simulink model "multiRobotSoccer"  (R2022b)
settings: Solver=FixedStepAuto  StartTime=0.0  StopTime=inf  FixedStep=sampleTime  RelTol=1e-3
PreLoadFcn:
  | robotSoccerParams;
values from neighbouring files (symbols this model uses):
  angThresh = pi/16    (= 0.196349540849)    [robotSoccerParams.m]
  attackerKickSpeed = 3    [robotSoccerParams.m]
  attackerMaxGoalDist = 10    [robotSoccerParams.m]
  attackerMinGoalDist = 5    [robotSoccerParams.m]
  awayGoalPosition = [fieldLimitsX(2) mean(fieldLimitsY)]    [robotSoccerParams.m]
  ballAngleNoise = pi/24    (= 0.1308996939)    [robotSoccerParams.m]
  ballThresh = robotRadius + 0.3    (= 1.1)    [robotSoccerParams.m]
  ballVelNoise = 0.5    [robotSoccerParams.m]
  defenderAwayPoses = [82 28.5 pi ... (first row only)    [robotSoccerParams.m]
  defenderHomePoses = [10 28.5 0 ... (first row only)    [robotSoccerParams.m]
  defenderKickSpeed = 5    [robotSoccerParams.m]
  distThresh = 1    [robotSoccerParams.m]
  dribbleKickSpeed = 2    [robotSoccerParams.m]
  dribbleTime = 25    [robotSoccerParams.m]
  fieldCenter = [mean(fieldLimitsX) mean(fieldLimitsY)]    [robotSoccerParams.m]
  fieldLimitsX = [0 92]    [robotSoccerParams.m]
  fieldLimitsY = [0 47]    [robotSoccerParams.m]
  goalkeeperKickSpeed = 10    [robotSoccerParams.m]
  goalkeeperPoses = [ 2 23.5 0 ... (first row only)    [robotSoccerParams.m]
  goalPosts = [ 0 33 2 ... (first row only)    [robotSoccerParams.m]
  goalThresh = 20    [robotSoccerParams.m]
  homeGoalPosition = [fieldLimitsX(1) mean(fieldLimitsY)]    [robotSoccerParams.m]
  initBallPos = fieldCenter    [robotSoccerParams.m]
  initGameState = struct('possession',0,                         'state',GameState.InPlay,                         'score',[0;0])    [robotSoccerParams.m]
  numRobots = 8    [robotSoccerParams.m]
  objColors = [0 0.75 0; 1 0 0; 0 0 1]    [robotSoccerParams.m]
  objMarkers = 'o^^'    [robotSoccerParams.m]
  outOfBoundsDist = 2    [robotSoccerParams.m]
  robotDetectorMaxHits = 5    [robotSoccerParams.m]
  robotRadius = 0.8    [robotSoccerParams.m]
undefined symbols (not defined in the file or in its folder): DiscIntNeverNeededParam, ObjectType
libraries: soccerRobotLib x8
(part 2 of 2)

== stateflow chart multiRobotSoccer/Robot Behavior/For Each Subsystem (Iterates through all robots)/SoccerBehavior ==
  settings: updateMethod=DISCRETE  sampleTime=sampleTime
  state ExecuteBehavior [parallel]
    en,du:
    prevRole = behavior.role;
    settings: executionOrder=1
    state Attack
      % Attack logic: Go to the ball, carry it near the goal, and shoot!
      en:
      if behavior.team == 1
      goalPose = [awayGoalPosition';0];
      else
      goalPose = [homeGoalPosition';pi];
      end
      state GoToBall
        en:
        commands.action = RobotAction.HoldBall;
        en,du:
        [ballRange,ballAngle] = detectBall(sensors.detections);
        commands.robotVelocity = trackDetection(ballRange,ballAngle);
      state KickBall
        en:
        commands.action = RobotAction.KickBall;
        commands.robotVelocity = [0;0;0];
        commands.ballVelocity = attackerKickSpeed;
      state GoToGoal
        en:
        commands.action = RobotAction.HoldBall;
        en,du:
        [goalDistance,goalAngle] = calcBearing(goalPose);
        commands.robotVelocity = goToPose(goalPose);
      state Dribble
        %Dribble the ball if held for too long
        en:
        commands.action = RobotAction.KickBall;
        commands.ballVelocity = dribbleKickSpeed;
      state BackUp
        % Move out of goal if too close
        en:
        commands.action = RobotAction.HoldBall;
        en,du:
        commands.robotVelocity = goToPose([fieldCenter';pi/2]);
      (default) -> GoToBall
      GoToBall -> ExecuteBehavior.Attack.GoToGoal : [sensors.ballHeld]
      ExecuteBehavior.Attack.KickBall -> GoToBall : [after(1,sec)]
      ExecuteBehavior.Attack.GoToGoal -> ExecuteBehavior.Attack.KickBall [order 2] : [goalDistance <= goalThresh && ...
          |  abs(goalAngle) < angThresh]
      ExecuteBehavior.Attack.GoToGoal -> Dribble [order 3] : [after(dribbleTime,sec)]
      Dribble -> ExecuteBehavior.Attack.GoToGoal : [after(0.5,sec)]
      ExecuteBehavior.Attack.GoToGoal -> BackUp [order 1] : [abs(sensors.pose(1) - goalPose(1)) < ...
          | attackerMinGoalDist]
      BackUp -> ExecuteBehavior.Attack.GoToGoal : [abs(sensors.pose(1) - goalPose(1)) > ...
          | attackerMaxGoalDist]
    state Defend
      % Defense logic: If own team has ball possession, go to the goal. Else, chase after the ball.
      state DefensiveActions
        en,du:
        ballRange = detectBall(sensors.detections);
        state DefendGoal
          en:
          commands.action = RobotAction.HoldBall;
          goalPose = behavior.formationPose;
          en,du:
          commands.robotVelocity = goToPose(goalPose);
        state ChaseBall
          en,du:
          if behavior.possessingTeam == 0
          commands.action = RobotAction.HoldBall;
          else
          commands.action = RobotAction.DoNothing;
          end
          [ballRange,ballAngle] = detectBall(sensors.detections);
          commands.robotVelocity = trackDetection(ballRange,ballAngle);
        (default) -> ExecuteBehavior.Defend.DefensiveActions.DefendGoal
        ExecuteBehavior.Defend.DefensiveActions.ChaseBall -> ExecuteBehavior.Defend.DefensiveActions.DefendGoal : [behavior.possessingTeam == behavior.team]
        ExecuteBehavior.Defend.DefensiveActions.DefendGoal -> ExecuteBehavior.Defend.DefensiveActions.ChaseBall : [behavior.possessingTeam == 0 ...
            |  && distToOwnGoal < diff(fieldLimitsX)/2 && ...
            |  ballRange < diff(fieldLimitsX)/1.5 && ballRange > 0]
      state TurnToGoal
        en:
        if behavior.team == 1
        goalPose = [awayGoalPosition';0];
        else
        goalPose = [homeGoalPosition';pi];
        end
        en,du:
        commands.action = RobotAction.HoldBall;
        [commands.robotVelocity,isdone] = turnToPoint(goalPose);
      state KickBall
        en:
        commands.action = RobotAction.KickBall;
        commands.robotVelocity = [0;0;0];
        commands.ballVelocity = defenderKickSpeed;
      state dist = distToOwnGoal [function]
        (default) -> (junction 441)
        (junction 441) -> (junction 444) [order 1] : [behavior.team == 1]
        (junction 441) -> (junction 448) [order 2] : {dist = calcBearing(awayGoalPosition');}
        (junction 444) -> (junction 446) : {dist = calcBearing(homeGoalPosition');}
        (junction 446) -> (junction 448)
      (default) -> ExecuteBehavior.Defend.DefensiveActions
      ExecuteBehavior.Defend.DefensiveActions -> ExecuteBehavior.Defend.TurnToGoal : [sensors.ballHeld]
      ExecuteBehavior.Defend.TurnToGoal -> ExecuteBehavior.Defend.KickBall : [isdone || after(10,sec)]
      ExecuteBehavior.Defend.KickBall -> ExecuteBehavior.Defend.DefensiveActions : [after(1,sec)]
    state Defend1
      % Defense logic: If own team has ball possession, go to the goal. Else, chase after the ball.
      state DefensiveActions
        en,du:
        ballRange = detectBall(sensors.detections);
        state DefendGoal
          en:
          commands.action = RobotAction.HoldBall;
          goalPose = behavior.formationPose;
          en,du:
          if behavior.possessingTeam == 0
          commands.action = RobotAction.HoldBall;
          else
          commands.action = RobotAction.DoNothing;
          end
          [ballRange,ballAngle] = detectBall(sensors.detections);
          commands.robotVelocity = trackDetection(ballRange,ballAngle);
        state ChaseBall
          en,du:
          if behavior.possessingTeam == 0
          commands.action = RobotAction.HoldBall;
          else
          commands.action = RobotAction.DoNothing;
          end
          [ballRange,ballAngle] = detectBall(sensors.detections);
          commands.robotVelocity = trackDetection(ballRange,ballAngle);
        (default) -> ExecuteBehavior.Defend1.DefensiveActions.DefendGoal
        ExecuteBehavior.Defend1.DefensiveActions.ChaseBall -> ExecuteBehavior.Defend1.DefensiveActions.DefendGoal : [behavior.possessingTeam == behavior.team]
        ExecuteBehavior.Defend1.DefensiveActions.DefendGoal -> ExecuteBehavior.Defend1.DefensiveActions.ChaseBall : [behavior.possessingTeam == 0 ...
            |  && distToOwnGoal < diff(fieldLimitsX)/2 && ...
            |  ballRange < diff(fieldLimitsX)/1.5 && ballRange > 0]
      state TurnToGoal
        en:
        if behavior.team == 1
        goalPose = [awayGoalPosition';0];
        else
        goalPose = [homeGoalPosition';pi];
        end
        en,du:
        commands.action = RobotAction.HoldBall;
        [commands.robotVelocity,isdone] = turnToPoint(goalPose);
      state KickBall
        en:
        commands.action = RobotAction.KickBall;
        commands.robotVelocity = [0;0;0];
        commands.ballVelocity = defenderKickSpeed;
      state dist = distToOwnGoal [function]
        (default) -> (junction 545)
        (junction 545) -> (junction 546) [order 1] : [behavior.team == 1]
        (junction 545) -> (junction 547) [order 2] : {dist = calcBearing(awayGoalPosition');}
        (junction 546) -> (junction 548) : {dist = calcBearing(homeGoalPosition');}
        (junction 548) -> (junction 547)
      (default) -> ExecuteBehavior.Defend1.DefensiveActions
      ExecuteBehavior.Defend1.DefensiveActions -> ExecuteBehavior.Defend1.TurnToGoal : [sensors.ballHeld]
      ExecuteBehavior.Defend1.TurnToGoal -> ExecuteBehavior.Defend1.KickBall : [isdone || after(10,sec)]
      ExecuteBehavior.Defend1.KickBall -> ExecuteBehavior.Defend1.DefensiveActions : [after(1,sec)]
    state Goalkeep
      % Goalkeeper logic: Wait for the ball and try hold it if nearby. If the ball is held, kick it far away!
      en:
      goalPose = behavior.formationPose;
      state GoalkeeperActions
        en, du:
        [ballRange,ballAngle] = detectBall(sensors.detections);
        state TurnToBall
          en:
          commands.robotVelocity = [0;0;0];
          commands.action = RobotAction.HoldBall;
          en,du:
          if ballAngle > angThresh
          commands.robotVelocity(3) = 1;
          elseif ballAngle < -angThresh
          commands.robotVelocity(3) = -1;
          else
          commands.robotVelocity(3) = 0;
          end
        state GoToGoal
          en,du:
          [commands.robotVelocity,isdone] = goToPose(goalPose);
          commands.action = RobotAction.HoldBall;
        (default) -> ExecuteBehavior.Goalkeep.GoalkeeperActions.GoToGoal
        ExecuteBehavior.Goalkeep.GoalkeeperActions.GoToGoal -> TurnToBall : [isdone && ballRange > 0]
        TurnToBall -> ExecuteBehavior.Goalkeep.GoalkeeperActions.GoToGoal : [ballRange < 0]
      state TurnToCenterline
        en,du:
        commands.robotVelocity = ...
        goToPose([fieldCenter';0]);
      state KickBall
        en:
        commands.robotVelocity = [0;0;0];
        commands.action = RobotAction.KickBall;
        commands.ballVelocity = goalkeeperKickSpeed;
      (default) -> GoalkeeperActions
      GoalkeeperActions -> TurnToCenterline : [sensors.ballHeld]
      ExecuteBehavior.Goalkeep.KickBall -> GoalkeeperActions : [after(1,sec)]
      TurnToCenterline -> ExecuteBehavior.Goalkeep.KickBall : [after(3,sec)]
    state DoNothing
      % Do not move, and do not do anything with the ball.
      en:
      commands.action = RobotAction.DoNothing;
      commands.robotVelocity = [0;0;0];
    (default) -> (junction 348)
    ExecuteBehavior -> (junction 348) : [behavior.role ~= prevRole]
    (junction 348) -> Attack [order 1] : [behavior.role==Role.Attacker]
    (junction 348) -> (junction 354) [order 2]
    Defend -> Attack : [behavior.possessingTeam == ...
        | behavior.team]
    Attack -> Defend : [behavior.possessingTeam == ...
        |  opposingTeam]
    (junction 354) -> Defend1 [order 1] : [behavior.role==Role.Defender]
    (junction 354) -> (junction 358) [order 2]
    (junction 358) -> Goalkeep [order 1] : [behavior.role==Role.Goalkeeper]
    (junction 358) -> (junction 361) [order 2]
    (junction 361) -> DoNothing
  state AvoidRobots [parallel]
    % All robots not holding the ball should avoid other robots using data from their Robot Detector sensors
    en,du:
    for idx = 1:robotDetectorMaxHits
    robotRanges(idx) = sensors.robotDetections(idx,1);
    end
    robotRanges(robotRanges<=0) = inf;
    [minRange,minRangeIdx] = min(robotRanges);
    settings: executionOrder=2
    state NormalOperation
      % Do not modify original commands to robot
    state Avoid
      en,du:
      % Move backwards and turn away from the commanded direction
      commands.robotVelocity(1) = -1;
      commands.robotVelocity(3) = -sign(sensors.robotDetections(minRangeIdx,2));
    (default) -> NormalOperation
    NormalOperation -> Avoid : [~sensors.ballHeld && ...
        | minRange < 3 && ~outOfBounds]
    Avoid -> NormalOperation : [after(1,sec) && ...
        | (~sensors.ballHeld || minRange > 5)]
  state [dist,ang] = calcBearing(goal) [function]
    (default) -> (junction 194) : % Calculate distance and angle to location
        | {
        | err = goal(1:2) - sensors.pose(1:2);
        | dist = norm(err);
        | ang = angdiff(sensors.pose(3),atan2(err(2),err(1)));
        | }
  state vel = trackDetection(dist,ang) [function]
    note: Uses range and bearing to track an object
    (default) -> (junction 321) : {
        | vel = [0;0;0];
        | }
    (junction 321) -> (junction 322) [order 1] : % Turn in place
        | % if no detection
        | [dist < 0]
    (junction 322) -> (junction 324) : {vel(3) = 1;}
    (junction 321) -> (junction 225) [order 2]
    (junction 225) -> (junction 229) [order 1] : % Forward speed
        | [dist > distThresh]
    (junction 225) -> (junction 231) [order 2]
    (junction 229) -> (junction 228) : {vel(1) = 1;}
    (junction 228) -> (junction 231)
    (junction 231) -> (junction 157)
    (junction 157) -> (junction 163) [order 1] : % Turning speed
        | [ang > angThresh]
    (junction 157) -> (junction 165) [order 2]
    (junction 163) -> (junction 172) : {vel(3) = 1;}
    (junction 165) -> (junction 167) [order 1] : [ang < -angThresh]
    (junction 165) -> (junction 162) [order 2]
    (junction 167) -> (junction 170) : {vel(3) = -1;}
    (junction 324) -> (junction 162)
    (junction 170) -> (junction 162)
    (junction 172) -> (junction 170)
  state [vel,done] = goToPose(goal) [function]
    note: Tracks a position. Once reached, the robot will turn in place until a reference angle is met.
    (default) -> (junction 247) : {
        | vel = [0;0;0];
        | [goalDist,goalAng] = calcBearing(goal(1:2));
        | trackAng = angdiff(sensors.pose(3),goal(3));
        | }
    (junction 247) -> (junction 248) [order 1] : % Track the position if outside the distance threshold
        | [goalDist > distThresh]
    (junction 247) -> (junction 299) [order 2] : % Else, turn in place until the angular reference is met
    (junction 248) -> (junction 280) : {vel = trackDetection(goalDist,goalAng);}
    (junction 299) -> (junction 300) [order 1] : [trackAng > angThresh]
    (junction 299) -> (junction 303) [order 2]
    (junction 300) -> (junction 284) : {vel(3) = 1;}
    (junction 303) -> (junction 305) [order 1] : [trackAng < -angThresh]
    (junction 303) -> (junction 310) [order 2]
    (junction 305) -> (junction 307) : {vel(3) = -1;}
    (junction 307) -> (junction 310)
    (junction 284) -> (junction 307)
    (junction 280) -> (junction 284)
    (junction 310) -> (junction 410) : {done = (goalDist <= distThresh) && (abs(trackAng) <= angThresh);}
  state [vel,done] = turnToPoint(goal) [function]
    note: Tracks a position. Once reached, the robot will turn in place until a reference angle is met.
    (default) -> (junction 375) : % Turn in place until the angular reference is met
        | {
        | done = false;
        | vel = [0;0;0];
        | [goalDist,goalAng] = calcBearing(goal(1:2));
        | }
    (junction 375) -> (junction 376) [order 1] : [goalAng > angThresh]
    (junction 375) -> (junction 377) [order 2]
    (junction 376) -> (junction 381) : {vel(3) = 1;}
    (junction 377) -> (junction 378) [order 1] : [goalAng < -angThresh]
    (junction 377) -> (junction 379) [order 2] : {done = true;}
    (junction 378) -> (junction 380) : {vel(3) = -1;}
    (junction 380) -> (junction 379)
    (junction 381) -> (junction 380)
  state flag = outOfBounds [function]
    note: Check whether a robot is out of bounds given a specified tolerance.
    (default) -> (junction 462) : {
        | flag = sensors.pose(1) <= fieldLimitsX(1)+outOfBoundsDist || ...
        |           sensors.pose(1) >= fieldLimitsX(2)-outOfBoundsDist || ...
        |           sensors.pose(2) <= fieldLimitsY(1)+outOfBoundsDist || ...
        |           sensors.pose(2) >= fieldLimitsY(2)-outOfBoundsDist;
        | }
  state team = opposingTeam [function]
    note: Convenience function that returns the number of the opposing team of a specific robot.
    (default) -> (junction 506)
    (junction 506) -> (junction 507) [order 1] : [behavior.team == 1]
    (junction 507) -> (junction 509) : {team = 2;}
    (junction 506) -> (junction 508) [order 2] : {team = 1;}
    (junction 509) -> (junction 508)
  data: dist function_output; dist function_output; goal function_input; dist function_output; ang function_output; dist function_input; ang function_input; vel function_output; vel function_output; done function_output; goal function_input; goal function_input; vel function_output; done function_output; flag function_output; team function_output; sensors input Bus: RobotSensorBus; behavior input; commands output Bus: RobotCommandBus; ballAngle local; ballRange local; goalPose local; distThresh parameter; goalThresh parameter; angThresh parameter; idx local =1; prevRole local =Role.None; isdone local =false; goalDistance local =0; goalAngle local =0; robotDetectorMaxHits parameter; homeGoalPosition parameter; awayGoalPosition parameter; fieldLimitsX parameter; fieldCenter parameter; fieldLimitsY parameter; minRangeIdx local; minRange local; robotRanges local =zeros(robotDetectorMaxHits,1); goalkeeperKickSpeed parameter; defenderKickSpeed parameter; attackerKickSpeed parameter; attackerMinGoalDist parameter; attackerMaxGoalDist parameter; dribbleKickSpeed parameter; dribbleTime parameter; outOfBoundsDist parameter double

== matlab function multiRobotSoccer/Soccer Field/World/Visualize ==
  data: visuals input; poses input; waypts input; numRobots parameter; ranges input; objs input; objDetParams input; robotDetParams input; plotSensorLines parameter; showRobotIds parameter
function visualizeWaypointsAndObjects(visuals,poses,waypts,numRobots,ranges,objs, ...
                                      objDetParams,robotDetParams,plotSensorLines, showRobotIds)

    coder.extrinsic('internal.multiRobotVizWorld')
    internal.multiRobotVizWorld(numRobots,visuals,poses,waypts,ranges,objs, ... 
                                objDetParams,robotDetParams,showRobotIds,plotSensorLines);

end
